simulink subsystem "Piero"  (R2023b)
settings: Solver=VariableStepAuto  StartTime=0.0  StopTime=10.0  RelTol=1e-3
settings Model: Creator=manu_  LastModifiedBy=manu_

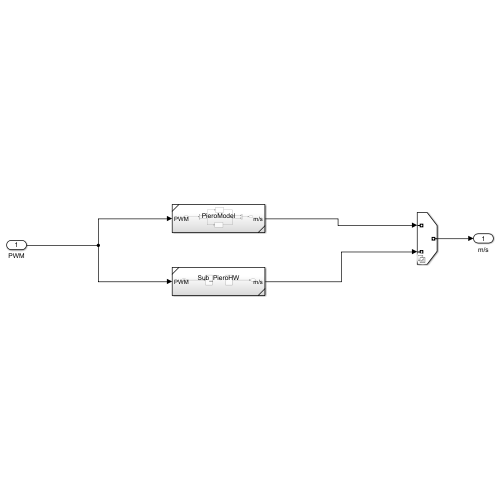
[thumbnail: Simulink's stored preview of the top-level diagram]
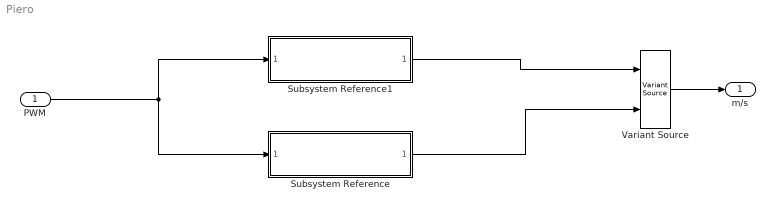
== system Piero ==
  PWM : Inport
  Subsystem Reference : Subsystem  ReferencedSubsystem=Sub_PieroHW
  Subsystem Reference1 : Subsystem  ReferencedSubsystem=PieroModel
  Variant Source : VariantSource  VariantControlMode=sim codegen switching
  m/s : Outport
  wires:
  Variant Source/1 -> m/s/1
  PWM/1 -> Subsystem Reference1/1, Subsystem Reference/1
  Subsystem Reference1/1 -> Variant Source/1
  Subsystem Reference/1 -> Variant Source/2
